simulink model "second"  (R2023b)
settings: Solver=FixedStepAuto  StartTime=0.0  StopTime=15  FixedStep=0.01  RelTol=1e-3
undefined symbols (not defined in the file): A, C, L, L1, L2, L3, x0, x1, xi
libraries: simulink x8
settings Model: Creator=evdokiiagalkina  LastModifiedBy=evdokiiagalkina

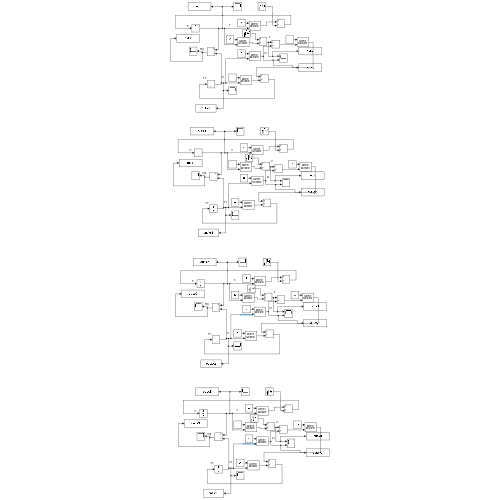
[thumbnail: Simulink's stored preview of the top-level diagram]
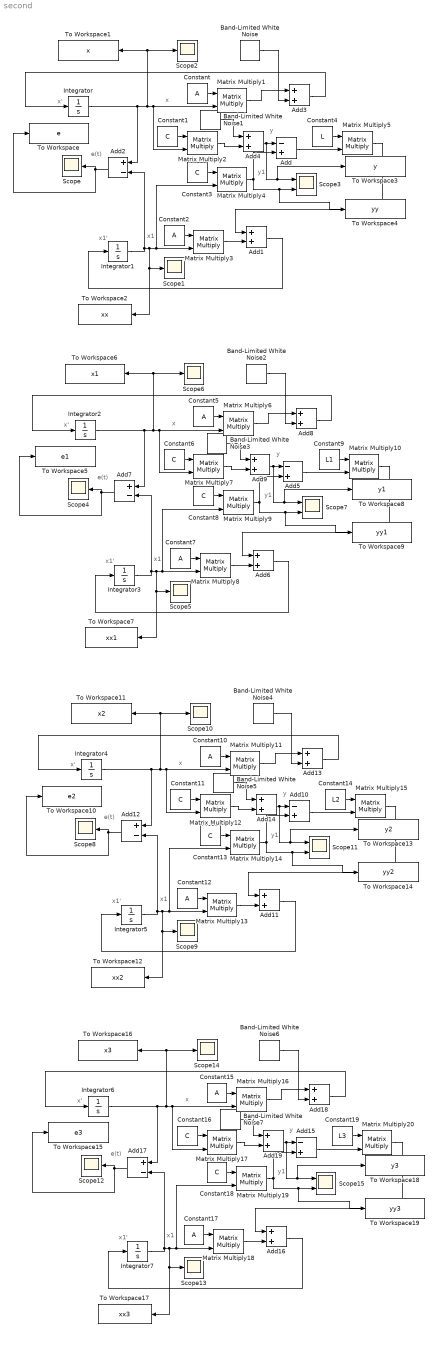
== system second ==
  note: x
  note: y
  note: x1'
  note: e(t)
  note: x'
  note: x1
  note: y1
  note: e(t)
  note: x1
  note: y1
  note: x
  note: x1'
  note: y
  note: x'
  note: e(t)
  note: x1
  note: y1
  note: x
  note: x1'
  note: y
  note: x'
  note: e(t)
  note: x1
  note: y1
  note: x
  note: x1'
  note: y
  note: x'
  Add{,5,10,15} (4 alike) : Sum  Inputs=-+
  Add{1,3..4,6,8..9,11,13..14,16,18..19} (12 alike) : Sum
  Add{2,7,12,17} (4 alike) : Sum  Inputs=+-
  Band-Limited White Noise{,2,4,6} (4 alike) : simulink/Sources/Band-Limited White Noise  Cov=[fi]  Ts=0.1  seed=[23341]
  Band-Limited White Noise{1,3,5,7} (4 alike) : simulink/Sources/Band-Limited White Noise  Cov=[xi]  Ts=0.1  seed=[23341]
  Constant{,2,5,7,10,12,15,17} (8 alike) : Constant  Value=A  VectorParams1D=off
  Constant{1,3,6,8,11,13,16,18} (8 alike) : Constant  Value=C  VectorParams1D=off
  Constant14 : Constant  Value=L2  VectorParams1D=off
  Constant19 : Constant  Value=L3  VectorParams1D=off
  Constant4 : Constant  Value=L  VectorParams1D=off
  Constant9 : Constant  Value=L1  VectorParams1D=off
  Integrator{,2,4,6} (4 alike) : Integrator  InitialCondition=x0
  Integrator{1,3,5,7} (4 alike) : Integrator  InitialCondition=x1
  Matrix Multiply{1..20} (20 alike) : Product  Multiplication=Matrix(*)
  Scope{,1..2,4..6,8..10,12..14} (12 alike) : Scope
  Scope{3,7,11,15} (4 alike) : Scope  NumInputPorts=2
  To Workspace : ToWorkspace  VariableName=e  SaveFormat=Timeseries  SampleTime=-1
  To Workspace1 : ToWorkspace  VariableName=x  SaveFormat=Timeseries  SampleTime=-1
  To Workspace10 : ToWorkspace  VariableName=e2  SaveFormat=Timeseries  SampleTime=-1
  To Workspace11 : ToWorkspace  VariableName=x2  SaveFormat=Timeseries  SampleTime=-1
  To Workspace12 : ToWorkspace  VariableName=xx2  SaveFormat=Timeseries  SampleTime=-1
  To Workspace13 : ToWorkspace  VariableName=y2  SaveFormat=Timeseries  SampleTime=-1
  To Workspace14 : ToWorkspace  VariableName=yy2  SaveFormat=Timeseries  SampleTime=-1
  To Workspace15 : ToWorkspace  VariableName=e3  SaveFormat=Timeseries  SampleTime=-1
  To Workspace16 : ToWorkspace  VariableName=x3  SaveFormat=Timeseries  SampleTime=-1
  To Workspace17 : ToWorkspace  VariableName=xx3  SaveFormat=Timeseries  SampleTime=-1
  To Workspace18 : ToWorkspace  VariableName=y3  SaveFormat=Timeseries  SampleTime=-1
  To Workspace19 : ToWorkspace  VariableName=yy3  SaveFormat=Timeseries  SampleTime=-1
  To Workspace2 : ToWorkspace  VariableName=xx  SaveFormat=Timeseries  SampleTime=-1
  To Workspace3 : ToWorkspace  VariableName=y  SaveFormat=Timeseries  SampleTime=-1
  To Workspace4 : ToWorkspace  VariableName=yy  SaveFormat=Timeseries  SampleTime=-1
  To Workspace5 : ToWorkspace  VariableName=e1  SaveFormat=Timeseries  SampleTime=-1
  To Workspace6 : ToWorkspace  VariableName=x1  SaveFormat=Timeseries  SampleTime=-1
  To Workspace7 : ToWorkspace  VariableName=xx1  SaveFormat=Timeseries  SampleTime=-1
  To Workspace8 : ToWorkspace  VariableName=y1  SaveFormat=Timeseries  SampleTime=-1
  To Workspace9 : ToWorkspace  VariableName=yy1  SaveFormat=Timeseries  SampleTime=-1
  wires:
  Constant2/1 -> Matrix Multiply3/1
  Matrix Multiply5/1 -> Add1/1
  Constant1/1 -> Matrix Multiply2/1
  Constant/1 -> Matrix Multiply1/1
  Add/1 -> Matrix Multiply5/2
  Integrator1/1 -> Add2/2, Scope1/1, To Workspace2/1, Matrix Multiply3/2, Matrix Multiply4/2
  Matrix Multiply4/1 -> Add/2, To Workspace4/1, Scope3/2
  Add1/1 -> Integrator1/1
  Matrix Multiply2/1 -> Add4/2
  Matrix Multiply3/1 -> Add1/2
  Integrator/1 -> Matrix Multiply1/2, Matrix Multiply2/2, Scope2/1, To Workspace1/1, Add2/1
  Constant4/1 -> Matrix Multiply5/1
  Add2/1 -> To Workspace/1, Scope/1
  Constant3/1 -> Matrix Multiply4/1
  Matrix Multiply1/1 -> Add3/1
  Band-Limited White Noise/1 -> Add3/2
  Add3/1 -> Integrator/1
  Band-Limited White Noise1/1 -> Add4/1
  Add4/1 -> To Workspace3/1, Scope3/1, Add/1
  Integrator3/1 -> Add7/2, Scope5/1, To Workspace7/1, Matrix Multiply8/2, Matrix Multiply9/2
  Matrix Multiply7/1 -> Add9/2
  Matrix Multiply9/1 -> Add5/2, To Workspace9/1, Scope7/2
  Add5/1 -> Matrix Multiply10/2
  Band-Limited White Noise3/1 -> Add9/1
  Matrix Multiply10/1 -> Add6/1
  Constant8/1 -> Matrix Multiply9/1
  Matrix Multiply8/1 -> Add6/2
  Constant5/1 -> Matrix Multiply6/1
  Integrator2/1 -> Matrix Multiply6/2, Matrix Multiply7/2, Scope6/1, To Workspace6/1, Add7/1
  Add8/1 -> Integrator2/1
  Add6/1 -> Integrator3/1
  Add9/1 -> To Workspace8/1, Scope7/1, Add5/1
  Add7/1 -> To Workspace5/1, Scope4/1
  Constant7/1 -> Matrix Multiply8/1
  Constant6/1 -> Matrix Multiply7/1
  Matrix Multiply6/1 -> Add8/1
  Band-Limited White Noise2/1 -> Add8/2
  Constant9/1 -> Matrix Multiply10/1
  Integrator5/1 -> Add12/2, Scope9/1, To Workspace12/1, Matrix Multiply13/2, Matrix Multiply14/2
  Matrix Multiply12/1 -> Add14/2
  Matrix Multiply14/1 -> Add10/2, To Workspace14/1, Scope11/2
  Add10/1 -> Matrix Multiply15/2
  Band-Limited White Noise5/1 -> Add14/1
  Matrix Multiply15/1 -> Add11/1
  Constant13/1 -> Matrix Multiply14/1
  Matrix Multiply13/1 -> Add11/2
  Constant10/1 -> Matrix Multiply11/1
  Integrator4/1 -> Matrix Multiply11/2, Matrix Multiply12/2, Scope10/1, To Workspace11/1, Add12/1
  Add13/1 -> Integrator4/1
  Add11/1 -> Integrator5/1
  Add14/1 -> To Workspace13/1, Scope11/1, Add10/1
  Add12/1 -> To Workspace10/1, Scope8/1
  Constant12/1 -> Matrix Multiply13/1
  Constant11/1 -> Matrix Multiply12/1
  Matrix Multiply11/1 -> Add13/1
  Band-Limited White Noise4/1 -> Add13/2
  Constant14/1 -> Matrix Multiply15/1
  Integrator7/1 -> Add17/2, Scope13/1, To Workspace17/1, Matrix Multiply18/2, Matrix Multiply19/2
  Matrix Multiply17/1 -> Add19/2
  Matrix Multiply19/1 -> Add15/2, To Workspace19/1, Scope15/2
  Add15/1 -> Matrix Multiply20/2
  Band-Limited White Noise7/1 -> Add19/1
  Matrix Multiply20/1 -> Add16/1
  Constant18/1 -> Matrix Multiply19/1
  Matrix Multiply18/1 -> Add16/2
  Constant15/1 -> Matrix Multiply16/1
  Integrator6/1 -> Matrix Multiply16/2, Matrix Multiply17/2, Scope14/1, To Workspace16/1, Add17/1
  Add18/1 -> Integrator6/1
  Add16/1 -> Integrator7/1
  Add19/1 -> To Workspace18/1, Scope15/1, Add15/1
  Add17/1 -> To Workspace15/1, Scope12/1
  Constant17/1 -> Matrix Multiply18/1
  Constant16/1 -> Matrix Multiply17/1
  Matrix Multiply16/1 -> Add18/1
  Band-Limited White Noise6/1 -> Add18/2
  Constant19/1 -> Matrix Multiply20/1
